simulink subsystem "CycleCount"  (R2022a)
settings: Solver=VariableStepAuto  StartTime=0.0  StopTime=10.0  RelTol=1e-3
settings Model: Creator=mateu  LastModifiedBy=mateu

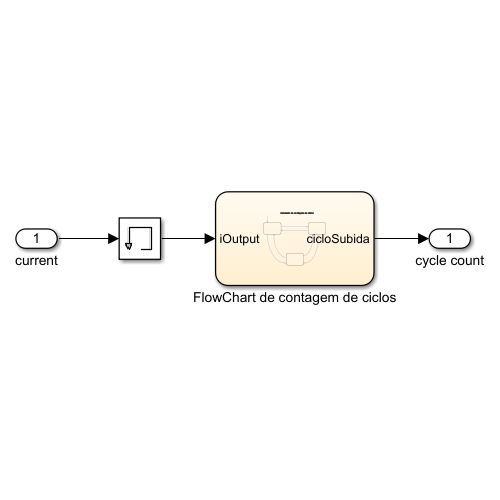
[thumbnail: Simulink's stored preview of the top-level diagram]
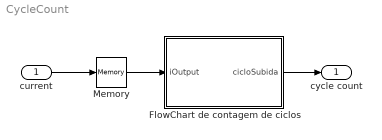
== system CycleCount ==
  current : Inport
  FlowChart de contagem de ciclos : Stateflow chart  TreatAsAtomicUnit=on
  Memory : Memory
  cycle count : Outport
  wires:
  Memory/1 -> FlowChart de contagem de ciclos/1(iOutput)
  current/1 -> Memory/1
  FlowChart de contagem de ciclos/1(cicloSubida) -> cycle count/1

== stateflow chart CycleCount/FlowChart de contagem de ciclos ==
  note: Automato de contagem de ciclos
  state Respouso
  state Descarregando
  state Carregando
  (default) -> Respouso
  Respouso -> Descarregando [order 1] : [iOutput<0]
  Descarregando -> Respouso [order 1] : [iOutput==0]
  Respouso -> Carregando [order 2] : [iOutput>0]{cicloSubida = cicloSubida + 1;}
  Carregando -> Respouso [order 2] : [iOutput==0]
  Carregando -> Descarregando [order 1] : [iOutput<0]
  Descarregando -> Carregando [order 2] : [iOutput>0]{cicloSubida = cicloSubida + 1;}
  data: cicloSubida output =-1; iOutput input
